simulink model "cstr_modelTest"  (R2022b)
settings: Solver=ode3  StartTime=0.0  StopTime=t(end)  FixedStep=ts  RelTol=1e-3  EnableMultiTasking=on
model workspace (MATLAB code in the model file):
  | % CSTR Initialization
  | % Parameters
  | alpha = 30.828;
  | delta = 3.556e-4;
  | Hab = 4.2;
  | beta = 86.688;
  | gamma = 0.1;
  | Hbc = -11;
  | cin = 5.1e3;
  | Tin = 104.9;
  | Had = -41.85;
  | T_k0 = 107.7; %
  | E1 = 9758.3;
  | k10 = 1.287e12;
  | E2 = 8560;
  | k20 = 9.043e6;
  | 
  | % Initial Conditions
  | cA0 = 0;
  | cB0 = 0;
  | Tr0 = 105;
  | Tj0 = 105;
  | 
  | x0 = [cA0;cB0;Tr0;Tj0];
  | 
  | ts = 1e-2;
  | t = 0:ts:1.8;
  | t = t';
settings Model: Creator=abp412  LastModifiedBy=Enrico
settings SolverCC: AlgebraicLoopSolver=TrustRegion
settings DataIOCC: LoadExternalInput=on  SaveFormat=Array  SignalLogging=off  DSMLogging=off
settings OptimizationCC: DefaultParameterBehavior=Inlined  ReuseModelBlockBuffer=on  ExpressionDepthLimit=2147483647  LifeSpan=inf
settings DebuggingCC: UnderspecifiedInitializationDetection=Classic  MergeDetectMultiDrivingBlocksExec=none  SolverPrmCheckMsg=warning  UnconnectedInputMsg=warning  UnconnectedOutputMsg=warning  UnconnectedLineMsg=warning  StateNameClashWarn=warning  SFUnexpectedBacktrackingDiag=warning  SFNoUnconditionalDefaultTransitionDiag=warning  SFExecutionAtInitializationDiag=none  ArithmeticOperatorsInVariantConditions=warning
settings HardwareCC: ProdBitPerPointer=32  ProdBitPerSizeT=32  ProdBitPerPtrDiffT=32  ProdLargestAtomicFloat=None  ProdIntDivRoundTo=Undefined  ProdEndianess=Unspecified  ProdWordSize=32  ProdHWDeviceType=32-bit Generic
settings ModelReferenceCC: EnableRefExpFcnMdlSchedulingChecks=on  PropagateSignalLabelsOutOfModel=off
settings SFSimCC: SimUseLocalCustomCode=off  CustomCodeUndefinedFunction=UseInterfaceOnly
settings RTWCC: RTWUseLocalCustomCode=off
settings CodeAppCC: StateflowObjectComments=on
settings GRTTargetCC: TargetLangStandard=C89/C90 (ANSI)
settings ConfigComp: CovMetricSettings=dw  CovSaveCumulativeToWorkspaceVar=on  CovSaveSingleToWorkspaceVar=on  CovExternalEMLEnable=off

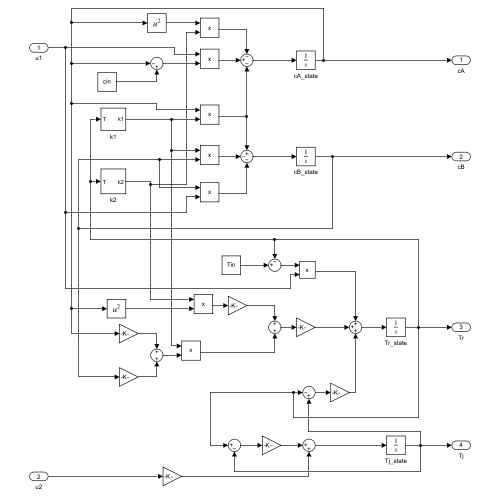
[thumbnail: Simulink's stored preview of the top-level diagram]
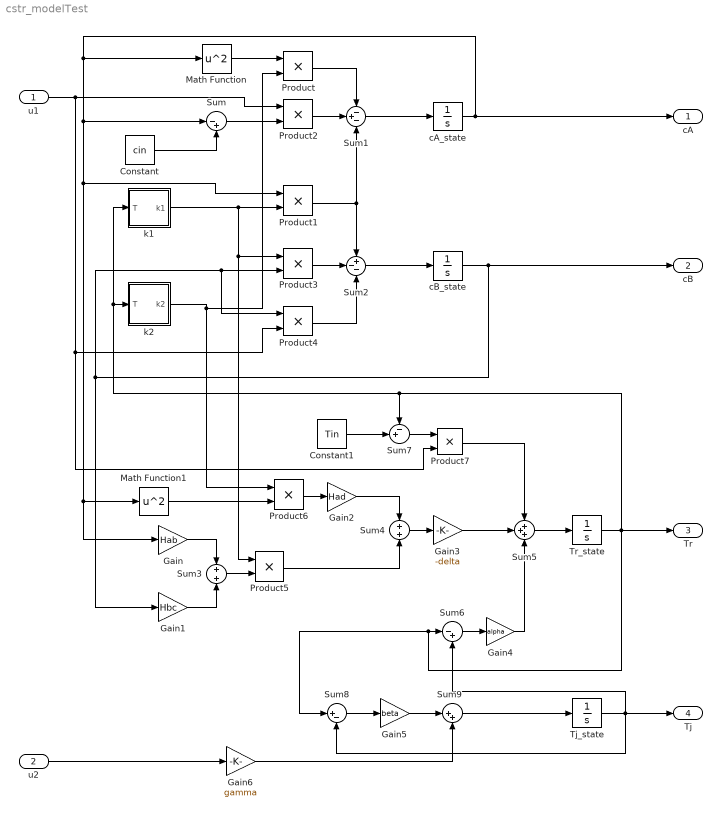
== system cstr_modelTest ==
  u1 : Inport
  u2 : Inport  Port=2
  Constant : Constant  Value=cin
  Constant1 : Constant  Value=Tin
  Gain : Gain  Gain=Hab
  Gain1 : Gain  Gain=Hbc
  Gain2 : Gain  Gain=Had
  Gain3 : Gain  Gain=-delta
  Gain4 : Gain  Gain=alpha
  Gain5 : Gain  Gain=beta
  Gain6 : Gain  Gain=gamma
  Math Function : Math  Operator=square  SignedPower=on
  Math Function1 : Math  Operator=square  SignedPower=on
  Product{,1..7} (8 alike) : Product  RndMeth=Zero
  Sum : Sum  Inputs=|-+
  Sum1 : Sum  Inputs=-+-
  Sum2 : Sum  Inputs=+--
  Sum3 : Sum
  Sum4 : Sum
  Sum5 : Sum  Inputs=+++
  Sum6 : Sum  Inputs=|-+
  Sum7 : Sum  Inputs=-+|
  Sum8 : Sum  Inputs=|+-
  Sum9 : Sum  Inputs=|++
  Tj_state : Integrator  InitialCondition=Tj0
  Tr_state : Integrator  InitialCondition=Tr0
  cA_state : Integrator  InitialCondition=cA0
  cB_state : Integrator  InitialCondition=cB0
  k1 : Subsystem
  k2 : Subsystem
  cA : Outport
  cB : Outport  Port=2
  Tr : Outport  Port=3
  Tj : Outport  Port=4
  wires:
  Tr_state/1 -> Tr/1, Sum6/1, Sum8/1, Sum7/1, k1/1(T), k2/1(T)
  cA_state/1 -> Math Function/1, Sum/1, Product1/1, Math Function1/1, Gain/1, cA/1
  k1/1(k1) -> Product3/1, Product5/1, Product1/2
  k2/1(k2) -> Product6/1, Product/2
  Math Function/1 -> Product/1
  Constant/1 -> Sum/2
  Sum/1 -> Product2/2
  u1/1 -> Product7/2, Product4/2, Product2/1
  Product2/1 -> Sum1/2
  Product/1 -> Sum1/1
  Product1/1 -> Sum2/1, Sum1/3
  Sum1/1 -> cA_state/1
  cB_state/1 -> cB/1, Product3/2, Product4/1, Gain1/1
  Product3/1 -> Sum2/2
  Product4/1 -> Sum2/3
  Sum2/1 -> cB_state/1
  Gain/1 -> Sum3/1
  Gain1/1 -> Sum3/2
  Sum3/1 -> Product5/2
  Math Function1/1 -> Product6/2
  Product6/1 -> Gain2/1
  Gain2/1 -> Sum4/1
  Product5/1 -> Sum4/2
  Sum4/1 -> Gain3/1
  Gain3/1 -> Sum5/2
  Tj_state/1 -> Sum8/2, Tj/1, Sum6/2
  Sum6/1 -> Gain4/1
  Gain4/1 -> Sum5/3
  Sum5/1 -> Tr_state/1
  Constant1/1 -> Sum7/2
  Sum8/1 -> Gain5/1
  u2/1 -> Gain6/1
  Gain6/1 -> Sum9/2
  Gain5/1 -> Sum9/1
  Sum9/1 -> Tj_state/1
  Sum7/1 -> Product7/1
  Product7/1 -> Sum5/1

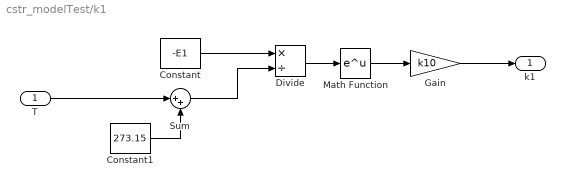
== system cstr_modelTest/k1 ==
  T : Inport
  Constant : Constant  Value=-E1
  Constant1 : Constant  Value=273.15
  Divide : Product  Inputs=*/
  Gain : Gain  Gain=k10
  Math Function : Math  SignedPower=on
  Sum : Sum  Inputs=|++
  k1 : Outport
  wires:
  Math Function/1 -> Gain/1
  Gain/1 -> k1/1
  Constant/1 -> Divide/1
  Constant1/1 -> Sum/2
  Sum/1 -> Divide/2
  T/1 -> Sum/1
  Divide/1 -> Math Function/1

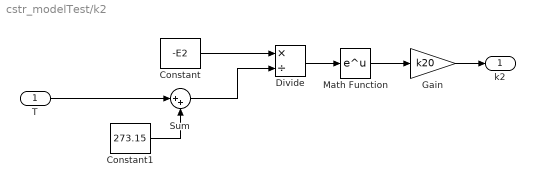
== system cstr_modelTest/k2 ==
  T : Inport
  Constant : Constant  Value=-E2
  Constant1 : Constant  Value=273.15
  Divide : Product  Inputs=*/
  Gain : Gain  Gain=k20
  Math Function : Math  SignedPower=on
  Sum : Sum  Inputs=|++
  k2 : Outport
  wires:
  Divide/1 -> Math Function/1
  T/1 -> Sum/1
  Sum/1 -> Divide/2
  Constant1/1 -> Sum/2
  Constant/1 -> Divide/1
  Gain/1 -> k2/1
  Math Function/1 -> Gain/1
